simulink library "testlib"  (Simulink 8.2)
settings: Solver=ode45  StartTime=0.0  StopTime=10.0  RelTol=1e-3
settings Model: Creator=Administrator  LastModifiedBy=Yuecheng

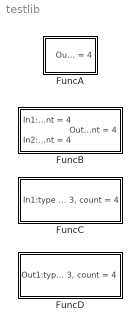
== system testlib ==
  FuncA : Subsystem
      mask Display: port_label('output', 1, '0')
  FuncB : Subsystem
  FuncC : Subsystem
  FuncD : Subsystem

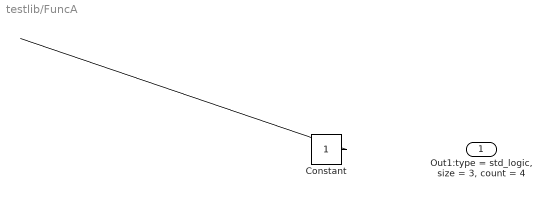
== system testlib/FuncA ==
  Constant : Constant
  "Out1:type = std_logic, size = 3, count = 4" : Outport
  wires:
  Constant/1 -> ?

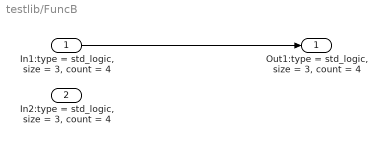
== system testlib/FuncB ==
  "In1:type = std_logic, size = 3, count = 4" : Inport
  "In2:type = std_logic, size = 3, count = 4" : Inport  Port=2
  "Out1:type = std_logic, size = 3, count = 4" : Outport
  wires:
  "In1:type = std_logic, size = 3, count = 4"/1 -> "Out1:type = std_logic, size = 3, count = 4"/1

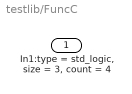
== system testlib/FuncC ==
  "In1:type = std_logic, size = 3, count = 4" : Inport

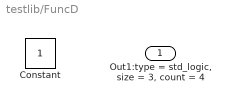
== system testlib/FuncD ==
  Constant : Constant
  "Out1:type = std_logic, size = 3, count = 4" : Outport
